simulink model "GGOV1_unitStepResponse"  (R2022a)
settings: Solver=VariableStepAuto  StartTime=0.0  StopTime=t_sim  RelTol=1e-3
undefined symbols (not defined in the file or in its folder): Ki, Kiload, Kp, Kpload, Kt, R, Tact, Tb, Tf, Tsa, Tsb
settings Model: Creator=jongoh  LastModifiedBy=jongoh

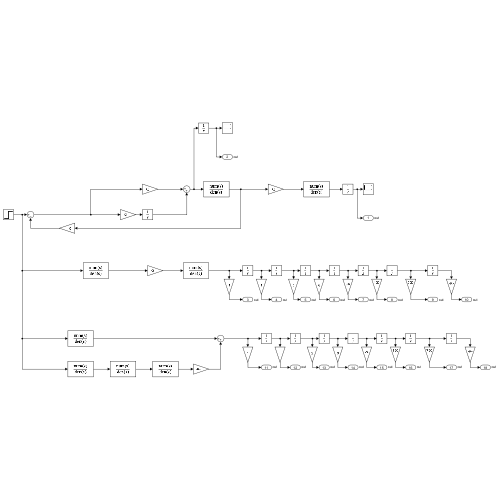
[thumbnail: Simulink's stored preview of the top-level diagram]
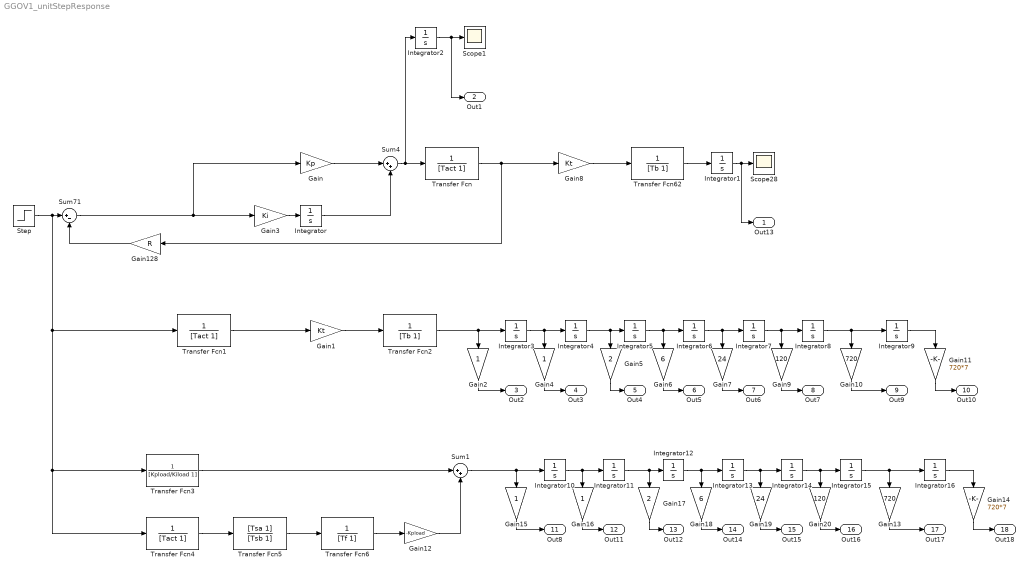
== system GGOV1_unitStepResponse ==
  Gain : Gain  Gain=Kp
  Gain1 : Gain  Gain=Kt
  Gain10 : Gain  Gain=720
  Gain11 : Gain  Gain=720*7
  Gain12 : Gain  Gain=-Kpload
  Gain128 : Gain  Gain=R
  Gain13 : Gain  Gain=720
  Gain14 : Gain  Gain=720*7
  Gain{2,4,15..16} (4 alike) : Gain
  Gain17 : Gain  Gain=2
  Gain18 : Gain  Gain=6
  Gain19 : Gain  Gain=24
  Gain20 : Gain  Gain=120
  Gain3 : Gain  Gain=Ki
  Gain5 : Gain  Gain=2
  Gain6 : Gain  Gain=6
  Gain7 : Gain  Gain=24
  Gain8 : Gain  Gain=Kt
  Gain9 : Gain  Gain=120
  Integrator{,1..16} (17 alike) : Integrator
  Scope1 : Scope
  Scope28 : Scope
  Step : Step  Time=0  SampleTime=0
  Sum1 : Sum  Inputs=|++
  Sum4 : Sum  Inputs=|++
  Sum71 : Sum  Inputs=|+-
  Transfer Fcn : TransferFcn  Denominator=[Tact 1]
  Transfer Fcn1 : TransferFcn  Denominator=[Tact 1]
  Transfer Fcn2 : TransferFcn  Denominator=[Tb 1]
  Transfer Fcn3 : TransferFcn  Denominator=[Kpload/Kiload 1]
  Transfer Fcn4 : TransferFcn  Denominator=[Tact 1]
  Transfer Fcn5 : TransferFcn  Numerator=[Tsa 1]  Denominator=[Tsb 1]
  Transfer Fcn6 : TransferFcn  Denominator=[Tf 1]
  Transfer Fcn62 : TransferFcn  Denominator=[Tb 1]
  Out13 : Outport  SignalName=out
  Out1 : Outport  Port=2  SignalName=out
  Out2 : Outport  Port=3  SignalName=out
  Out3 : Outport  Port=4  SignalName=out
  Out4 : Outport  Port=5  SignalName=out
  Out5 : Outport  Port=6  SignalName=out
  Out6 : Outport  Port=7  SignalName=out
  Out7 : Outport  Port=8  SignalName=out
  Out9 : Outport  Port=9  SignalName=out
  Out10 : Outport  Port=10  SignalName=out
  Out8 : Outport  Port=11  SignalName=out
  Out11 : Outport  Port=12  SignalName=out
  Out12 : Outport  Port=13  SignalName=out
  Out14 : Outport  Port=14  SignalName=out
  Out15 : Outport  Port=15  SignalName=out
  Out16 : Outport  Port=16  SignalName=out
  Out17 : Outport  Port=17  SignalName=out
  Out18 : Outport  Port=18  SignalName=out
  wires:
  Integrator1/1 -> Out13/1, Scope28/1
  Sum4/1 -> Integrator2/1, Transfer Fcn/1
  Transfer Fcn/1 -> Gain8/1, Gain128/1
  Gain128/1 -> Sum71/2
  Step/1 -> Transfer Fcn4/1, Transfer Fcn3/1, Transfer Fcn1/1, Sum71/1
  Transfer Fcn62/1 -> Integrator1/1
  Gain3/1 -> Integrator/1
  Sum71/1 -> Gain/1, Gain3/1
  Gain/1 -> Sum4/1
  Integrator/1 -> Sum4/2
  Gain8/1 -> Transfer Fcn62/1
  Integrator2/1 -> Out1/1, Scope1/1
  Transfer Fcn2/1 -> Gain2/1, Integrator3/1
  Gain1/1 -> Transfer Fcn2/1
  Transfer Fcn1/1 -> Gain1/1
  Integrator3/1 -> Gain4/1, Integrator4/1
  Integrator4/1 -> Gain5/1, Integrator5/1
  Integrator5/1 -> Gain6/1, Integrator6/1
  Integrator6/1 -> Gain7/1, Integrator7/1
  Integrator7/1 -> Gain9/1, Integrator8/1
  Integrator9/1 -> Gain11/1
  Integrator8/1 -> Gain10/1, Integrator9/1
  Gain2/1 -> Out2/1
  Gain4/1 -> Out3/1
  Gain5/1 -> Out4/1
  Gain6/1 -> Out5/1
  Gain7/1 -> Out6/1
  Gain9/1 -> Out7/1
  Gain10/1 -> Out9/1
  Gain11/1 -> Out10/1
  Transfer Fcn6/1 -> Gain12/1
  Transfer Fcn3/1 -> Sum1/1
  Gain12/1 -> Sum1/2
  Gain13/1 -> Out17/1
  Gain19/1 -> Out15/1
  Gain18/1 -> Out14/1
  Gain14/1 -> Out18/1
  Gain20/1 -> Out16/1
  Sum1/1 -> Gain15/1, Integrator10/1
  Integrator10/1 -> Gain16/1, Integrator11/1
  Integrator12/1 -> Gain18/1, Integrator13/1
  Gain15/1 -> Out8/1
  Integrator15/1 -> Gain13/1, Integrator16/1
  Integrator14/1 -> Gain20/1, Integrator15/1
  Gain17/1 -> Out12/1
  Gain16/1 -> Out11/1
  Integrator13/1 -> Gain19/1, Integrator14/1
  Integrator16/1 -> Gain14/1
  Integrator11/1 -> Gain17/1, Integrator12/1
  Transfer Fcn4/1 -> Transfer Fcn5/1
  Transfer Fcn5/1 -> Transfer Fcn6/1
